simulink model "modelofisicocompleto"  (R2017a)
settings: Solver=FixedStepAuto  StartTime=0.0  StopTime=inf  FixedStep=1e-3  MaxStep=1e-3  RelTol=1e-3
undefined symbols (not defined in the file): bac, baiz, bcx, bcy, Beqtran, Bheqd, bw, g, Kcy, ksac, ksaiz, ksiac, ksiaiz, Kw, lh0, Meq, Mheq, Rd, Rr, rt, rtd, tau, xl0, xt0, yl0, yt0
libraries: simulink x3, powerlib_meascontrol x2, vrlib x1
settings Model: SimulationMode=accelerator  Creator=tomas  LastModifiedBy=tomas
settings HardwareCC: ProdBitPerPointer=32  ProdBitPerSizeT=32  ProdBitPerPtrDiffT=32  ProdWordSize=32  ProdHWDeviceType=Intel->x86-32 (Windows32)

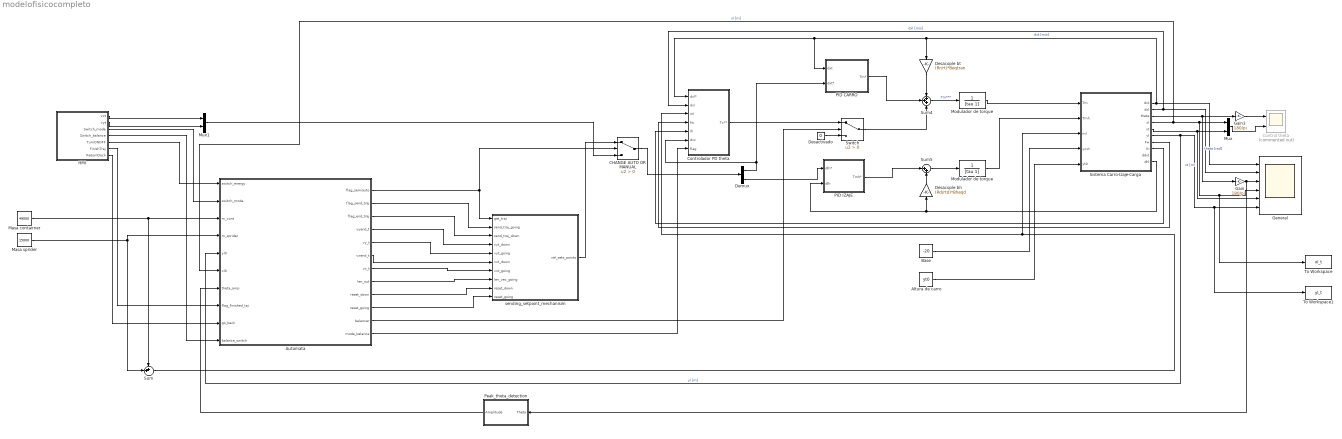
== system modelofisicocompleto ==
  Altura de carro : Constant  Value=yt0
  Automata : Stateflow chart  TreatAsAtomicUnit=on
  "Base " : Constant  Value=-20
  CHANGE AUTO OR MANUAL : Switch  Criteria=u2 > Threshold
  Control theta : Scope  Commented=on  NumInputPorts=2
  Controlador PD theta : Subsystem
  Demux : Demux  Outputs=2
  Desacople bh : Gain  Gain=(Rd/rtd)*Bheqd
  Desacople bt : Gain  Gain=(Rr/rt)*Beqtran
  Desactivado : Constant  Value=0
  Gain : Gain  Gain=180/pi
  Gain3 : Gain  Gain=180/pi
  General : Scope  NumInputPorts=6
  HMI : Subsystem
  Masa contairner : Constant  Value=49000
  Masa sprider : Constant  Value=15000
  Modulador de torque : TransferFcn  Denominator=[tau 1]
  "Modulador de torque  " : TransferFcn  Denominator=[tau 1]
  Mux : Mux  Inputs=2
  Mux1 : Mux  Inputs=2
  "PID CARRO " : Subsystem
  PID IZAJE : Subsystem
  Peak_theta_detection : Subsystem
  "Sistema Carro-Izaje-Carga " : Subsystem
  Sum : Sum  Inputs=++|
  Sum4 : Sum  Inputs=+++
  Sum5 : Sum  Inputs=|++
  Switch : Switch  Criteria=u2 > Threshold
  To Workspace : ToWorkspace  VariableName=xl_t  SampleTime=-1
  To Workspace1 : ToWorkspace  VariableName=yl_t  SampleTime=-1
  sending_setpoint_mechanisim : Subsystem
  wires:
  Sum4/1 -> "Modulador de torque  "/1  "Tm***"
  Desacople bt/1 -> Sum4/1
  Sum5/1 -> Modulador de torque/1
  Desacople bh/1 -> Sum5/2
  PID IZAJE/1("Tmh* ") -> Sum5/1
  Switch/1 -> Sum4/3
  Modulador de torque/1 -> "Sistema Carro-Izaje-Carga "/2(Tmh)
  "Base "/1 -> "Sistema Carro-Izaje-Carga "/4(ycxt)
  Altura de carro/1 -> "Sistema Carro-Izaje-Carga "/5(yt0)
  "Sistema Carro-Izaje-Carga "/1(dxt) -> Controlador PD theta/1(dxl*), "PID CARRO "/1(dxt), Desacople bt/1, General/1  "dxt [m/s]"
  "Sistema Carro-Izaje-Carga "/10(dhl) -> PID IZAJE/2(dlh), Desacople bh/1
  Controlador PD theta/1(Tc**) -> Switch/1
  Desactivado/1 -> Switch/3
  "Sistema Carro-Izaje-Carga "/8(lh) -> Controlador PD theta/5(lh)
  "Sistema Carro-Izaje-Carga "/7(Fw) -> Controlador PD theta/4(fw)
  Sum/1 -> Controlador PD theta/3(ml), "Sistema Carro-Izaje-Carga "/3(ml)
  "Sistema Carro-Izaje-Carga "/2(dxl) -> Controlador PD theta/2(dxl), General/2  "dxl [m/s]"
  Mux/1 -> Control theta/2
  "Sistema Carro-Izaje-Carga "/3(theta) -> Gain/1, Gain3/1  "theta [rad]"
  "Sistema Carro-Izaje-Carga "/4(xl) -> Automata/6(xl0), To Workspace/1, General/4, Mux/1  "xl [m]"
  "Sistema Carro-Izaje-Carga "/5(xt) -> General/5, Mux/2  "xt [m]"
  "Sistema Carro-Izaje-Carga "/6(yl) -> Automata/5(yl0), To Workspace1/1, General/6  "yl [m]"
  "Modulador de torque  "/1 -> "Sistema Carro-Izaje-Carga "/1(Tm)
  "PID CARRO "/1(Tm*) -> Sum4/2
  Gain/1 -> Peak_theta_detection/1(Theta), General/3
  Masa sprider/1 -> Automata/4(m_sprider), Sum/2
  Masa contairner/1 -> Sum/1, Automata/3(m_cont)
  Gain3/1 -> Control theta/1
  Automata/11(balancer) -> Switch/2
  HMI/4(Switch_balance) -> Automata/10(balance_switch)
  HMI/3(Switch_mode) -> Automata/2(switch_mode)
  HMI/1(vxt) -> Mux1/1
  HMI/2(vyt) -> Mux1/2
  Automata/1(flag_semiauto) -> CHANGE AUTO OR MANUAL/2, sending_setpoint_mechanisim/1(get_traj)
  CHANGE AUTO OR MANUAL/1 -> Demux/1
  Demux/1 -> Controlador PD theta/6(dxc), "PID CARRO "/2(dxt*)
  Demux/2 -> PID IZAJE/1(dlh*)
  Peak_theta_detection/1(Amplitude) -> Automata/7(theta_amp)
  Mux1/1 -> CHANGE AUTO OR MANUAL/3
  HMI/5(TurnONOFF) -> Automata/1(switch_energy)
  HMI/6(FinishTraj) -> Automata/8(flag_finished_taj)
  HMI/7(ReturnDock) -> Automata/9(go_back)
  Automata/2(flag_send_traj) -> sending_setpoint_mechanisim/2(send_traj_going)
  Automata/3(flag_end_traj) -> sending_setpoint_mechanisim/3(send_traj_down)
  sending_setpoint_mechanisim/1(vel_sets_points) -> CHANGE AUTO OR MANUAL/1
  Automata/7(vx_t) -> sending_setpoint_mechanisim/7(vxt_going)
  Automata/5(vy_t) -> sending_setpoint_mechanisim/5(vyt_going)
  Automata/4(vyend_t) -> sending_setpoint_mechanisim/4(vyt_down)
  Automata/6(vxend_t) -> sending_setpoint_mechanisim/6(vxt_down)
  Automata/8(len_out) -> sending_setpoint_mechanisim/8(len_vec_going)
  Automata/10(reset_going) -> sending_setpoint_mechanisim/10(reset_going)
  Automata/9(reset_down) -> sending_setpoint_mechanisim/9(reset_down)
  Automata/12(mode_balance) -> Controlador PD theta/7("flag ")

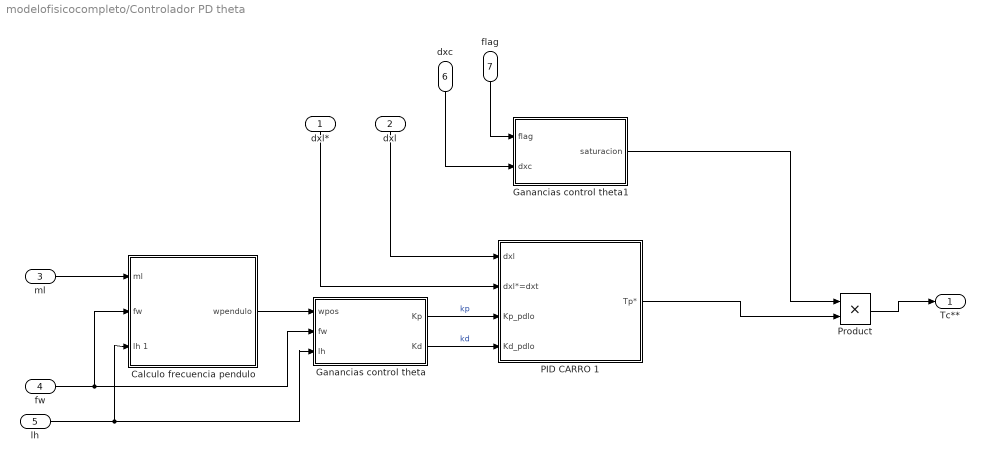
== system modelofisicocompleto/Controlador PD theta ==
  dxl* : Inport
  dxl : Inport  Port=2
  ml : Inport  Port=3
  fw : Inport  Port=4
  lh : Inport  Port=5
  dxc : Inport  Port=6
  "flag " : Inport  Port=7
  Calculo frecuencia pendulo : Subsystem
  Ganancias control theta : MATLAB Function  TreatAsAtomicUnit=on
  Ganancias control theta1 : MATLAB Function  TreatAsAtomicUnit=on
  PID CARRO 1 : Subsystem
  Product : Product
  Tc** : Outport
  wires:
  Calculo frecuencia pendulo/1("wpendulo ") -> Ganancias control theta/1(wpos)
  ml/1 -> Calculo frecuencia pendulo/1("ml ")
  Ganancias control theta/1(Kp) -> PID CARRO 1/3(Kp_pdlo)  "kp"
  Ganancias control theta/2(Kd) -> PID CARRO 1/4(Kd_pdlo)  "kd"
  dxl/1 -> PID CARRO 1/1(dxl)
  lh/1 -> Calculo frecuencia pendulo/3(lh 1), Ganancias control theta/3(lh)
  fw/1 -> Calculo frecuencia pendulo/2("fw "), Ganancias control theta/2(fw)
  dxl*/1 -> PID CARRO 1/2(dxl*=dxt)
  PID CARRO 1/1(Tp*) -> Product/2
  dxc/1 -> Ganancias control theta1/2(dxc)
  Ganancias control theta1/1(saturacion) -> Product/1
  Product/1 -> Tc**/1
  "flag "/1 -> Ganancias control theta1/1(flag)

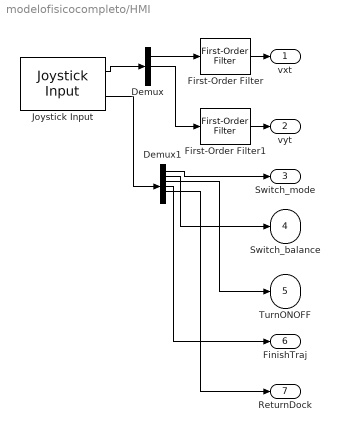
== system modelofisicocompleto/HMI ==
  Demux : Demux  Outputs=3
  Demux1 : Demux  Outputs=6
  First-Order Filter : powerlib_meascontrol/Filters/First-Order Filter  FilterType=Lowpass  Tc=10e-3  Ts=0  Initialize=off  Vac_Init=[0, 0, 60]  Vdc_Init=0  PlotResponse=off  FreqRange="[0,  200,  1]"
      settings: SourceProductName=Simscape Power Systems
  First-Order Filter1 : powerlib_meascontrol/Filters/First-Order Filter  FilterType=Lowpass  Tc=10e-3  Ts=0  Initialize=off  Vac_Init=[0, 0, 60]  Vdc_Init=0  PlotResponse=off  FreqRange="[0,  200,  1]"
      settings: SourceProductName=Simscape Power Systems
  Joystick Input : vrlib/Joystick Input  joyid=1  adjustports=on  forcefeed=off
      settings: SourceProductBaseCode=VR
  vxt : Outport
  vyt : Outport  Port=2
  Switch_mode : Outport  Port=3
  Switch_balance : Outport  Port=4
  TurnONOFF : Outport  Port=5
  FinishTraj : Outport  Port=6
  ReturnDock : Outport  Port=7
  wires:
  First-Order Filter1/1 -> vyt/1
  First-Order Filter/1 -> vxt/1
  Demux1/2 -> Switch_balance/1
  Joystick Input/2 -> Demux1/1
  Demux1/1 -> Switch_mode/1
  Joystick Input/1 -> Demux/1
  Demux/1 -> First-Order Filter/1
  Demux/2 -> First-Order Filter1/1
  Demux1/3 -> TurnONOFF/1
  Demux1/4 -> FinishTraj/1
  Demux1/5 -> ReturnDock/1

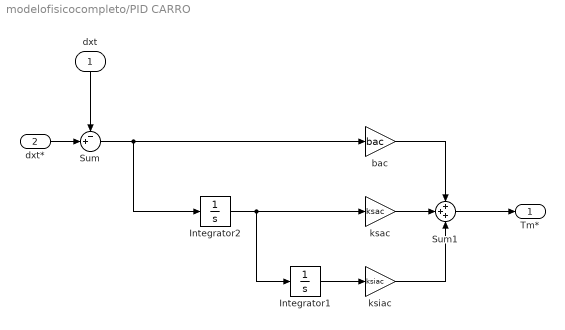
== system modelofisicocompleto/PID CARRO  ==
  dxt : Inport
  dxt* : Inport  Port=2
  Integrator1 : Integrator
  Integrator2 : Integrator
  Sum : Sum  Inputs=-+|
  Sum1 : Sum  Inputs=+++
  bac : Gain  Gain=bac
  ksac : Gain  Gain=ksac
  ksiac : Gain  Gain=ksiac
  Tm* : Outport
  wires:
  dxt*/1 -> Sum/2
  dxt/1 -> Sum/1
  Sum1/1 -> Tm*/1
  bac/1 -> Sum1/1
  ksac/1 -> Sum1/2
  Integrator1/1 -> ksiac/1
  ksiac/1 -> Sum1/3
  Sum/1 -> bac/1, Integrator2/1
  Integrator2/1 -> Integrator1/1, ksac/1

== system modelofisicocompleto/PID IZAJE ==
  dlh* : Inport
  dlh : Inport  Port=2
  Integrator1 : Integrator
  Integrator2 : Integrator
  Sum2 : Sum  Inputs=|+-
  Sum3 : Sum  Inputs=+++
  baiz : Gain  Gain=baiz
  ksaiz : Gain  Gain=ksaiz
  ksiaiz : Gain  Gain=ksiaiz
  "Tmh* " : Outport
  wires:
  dlh/1 -> Sum2/2
  Sum3/1 -> "Tmh* "/1
  ksaiz/1 -> Sum3/2
  Integrator1/1 -> ksiaiz/1
  baiz/1 -> Sum3/1
  ksiaiz/1 -> Sum3/3
  dlh*/1 -> Sum2/1
  Sum2/1 -> baiz/1, Integrator2/1
  Integrator2/1 -> Integrator1/1, ksaiz/1

== system modelofisicocompleto/Peak_theta_detection ==
  Theta : Inport
  Detect Decrease : simulink/Logic and Bit Operations/Detect Decrease  vinit=0.0  OutDataTypeStr=boolean
  Detect Rise Positive : simulink/Logic and Bit Operations/Detect Rise Positive  vinit=0  OutDataTypeStr=boolean
  MinMax Running Resettable : simulink/Math Operations/MinMax Running Resettable  Function=max  vinit=0.0
  Subsystem : Subsystem
  Amplitude : Outport
  wires:
  Theta/1 -> Detect Decrease/1, Detect Rise Positive/1, MinMax Running Resettable/1
  Subsystem/1(Out1) -> Amplitude/1
  MinMax Running Resettable/1 -> Subsystem/1(In1)
  Detect Rise Positive/1 -> MinMax Running Resettable/2
  Detect Decrease/1 -> Subsystem/Trigger

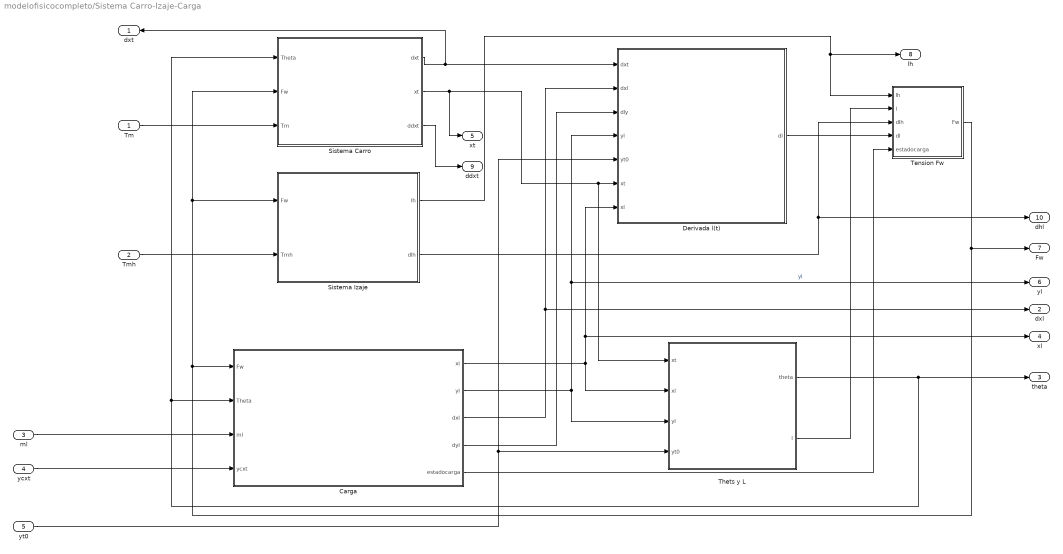
== system modelofisicocompleto/Sistema Carro-Izaje-Carga  ==
  Tm : Inport
  Tmh : Inport  Port=2
  ml : Inport  Port=3
  ycxt : Inport  Port=4
  yt0 : Inport  Port=5
  "Carga " : Subsystem
  Derivada l(t) : Subsystem
  Sistema Carro : Subsystem
  Sistema Izaje : Subsystem
  Tension Fw : Subsystem
  Thets y L : Subsystem
  dxt : Outport
  dxl : Outport  Port=2
  theta : Outport  Port=3
  xl : Outport  Port=4
  xt : Outport  Port=5
  yl : Outport  Port=6
  Fw : Outport  Port=7
  lh : Outport  Port=8
  ddxt : Outport  Port=9
  dhl : Outport  Port=10
  wires:
  Sistema Carro/2(xt) -> xt/1, Derivada l(t)/6(xt), Thets y L/1(xt)
  Sistema Carro/1("dxt ") -> dxt/1, Derivada l(t)/1(dxt)
  Sistema Izaje/1(lh) -> lh/1, Tension Fw/1(lh)
  Sistema Izaje/2(dlh) -> dhl/1, Tension Fw/3(dlh)
  "Carga "/2(yl) -> yl/1, Derivada l(t)/4(yl), Thets y L/3(yl)  "yl"
  "Carga "/3(dxl) -> dxl/1, Derivada l(t)/2(dxl)
  "Carga "/4(dyl) -> Derivada l(t)/3(dly)
  Derivada l(t)/1(dl) -> Tension Fw/4(dl)
  Thets y L/1("theta ") -> theta/1, Sistema Carro/1(Theta), "Carga "/2(Theta)
  ml/1 -> "Carga "/3(ml)
  ycxt/1 -> "Carga "/4(ycxt)
  "Carga "/5("estadocarga ") -> Tension Fw/5(estadocarga)
  Thets y L/2("l ") -> Tension Fw/2(l)
  Tm/1 -> Sistema Carro/3(Tm)
  Tmh/1 -> Sistema Izaje/2(Tmh)
  yt0/1 -> Derivada l(t)/5(yt0), Thets y L/4(yt0)
  "Carga "/1(xl) -> Derivada l(t)/7(xl), xl/1, Thets y L/2(xl)
  Tension Fw/1("Fw ") -> Fw/1, Sistema Carro/2(Fw), Sistema Izaje/1(Fw), "Carga "/1(Fw)
  Sistema Carro/3("ddxt ") -> ddxt/1

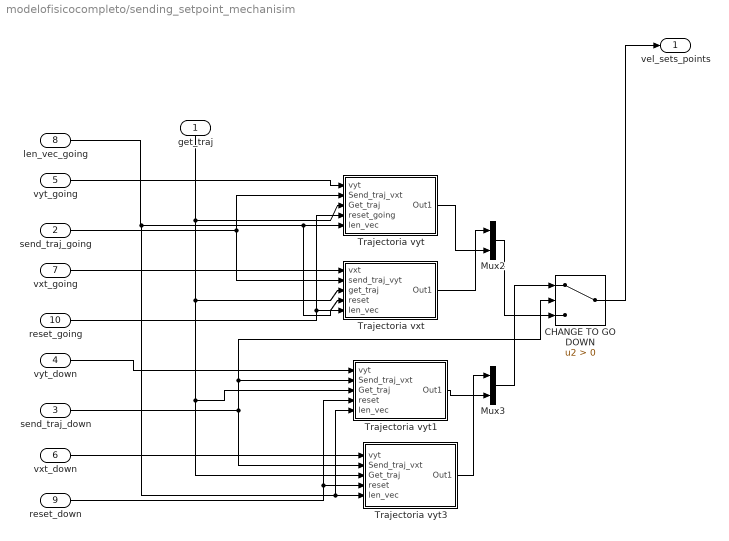
== system modelofisicocompleto/sending_setpoint_mechanisim ==
  get_traj : Inport
  send_traj_going : Inport  Port=2
  send_traj_down : Inport  Port=3
  vyt_down : Inport  Port=4
  vyt_going : Inport  Port=5
  vxt_down : Inport  Port=6
  vxt_going : Inport  Port=7
  len_vec_going : Inport  Port=8
  reset_down : Inport  Port=9
  reset_going : Inport  Port=10
  CHANGE TO GO DOWN : Switch  Criteria=u2 > Threshold
  Mux2 : Mux  Inputs=2
  Mux3 : Mux  Inputs=2
  Trajectoria vxt : Subsystem
  Trajectoria vyt : Subsystem
  Trajectoria vyt1 : Subsystem
  Trajectoria vyt3 : Subsystem
  vel_sets_points : Outport
  wires:
  get_traj/1 -> Trajectoria vyt3/3(Get_traj), Trajectoria vyt1/3(Get_traj), Trajectoria vxt/3("get_traj "), Trajectoria vyt/3(Get_traj)
  vyt_going/1 -> Trajectoria vyt/1("vyt ")
  Trajectoria vxt/1(Out1) -> Mux2/1
  Trajectoria vyt/1(Out1) -> Mux2/2
  vxt_going/1 -> Trajectoria vxt/1(vxt)
  send_traj_going/1 -> Trajectoria vxt/2(send_traj_vyt), Trajectoria vyt/2("Send_traj_vxt ")
  vyt_down/1 -> Trajectoria vyt1/1("vyt ")
  vxt_down/1 -> Trajectoria vyt3/1("vyt ")
  send_traj_down/1 -> Trajectoria vyt3/2("Send_traj_vxt "), Trajectoria vyt1/2("Send_traj_vxt "), CHANGE TO GO DOWN/2
  Trajectoria vyt1/1(Out1) -> Mux3/2
  Trajectoria vyt3/1(Out1) -> Mux3/1
  CHANGE TO GO DOWN/1 -> vel_sets_points/1
  Mux3/1 -> CHANGE TO GO DOWN/1
  Mux2/1 -> CHANGE TO GO DOWN/3
  reset_going/1 -> Trajectoria vxt/4(reset), Trajectoria vyt/4(reset_going)
  reset_down/1 -> Trajectoria vyt3/4(reset), Trajectoria vyt1/4(reset)
  len_vec_going/1 -> Trajectoria vyt3/5(len_vec), Trajectoria vyt1/5(len_vec), Trajectoria vxt/5(len_vec), Trajectoria vyt/5(len_vec)

== system modelofisicocompleto/Controlador PD theta/Calculo frecuencia pendulo ==
  "ml " : Inport
  "fw " : Inport  Port=2
  lh 1 : Inport  Port=3
  Abs : Abs
  Divide : Product  Inputs=*/
  Gain : Gain  Gain=80
  Product : Product
  Sqrt : Sqrt  OutputSignalType=complex  SaturateOnIntegerOverflow=on
  "wpendulo " : Outport
  wires:
  "fw "/1 -> Divide/1
  Divide/1 -> Sqrt/1
  lh 1/1 -> Product/2
  Product/1 -> Divide/2
  Sqrt/1 -> Abs/1
  "ml "/1 -> Product/1
  Abs/1 -> Gain/1
  Gain/1 -> "wpendulo "/1

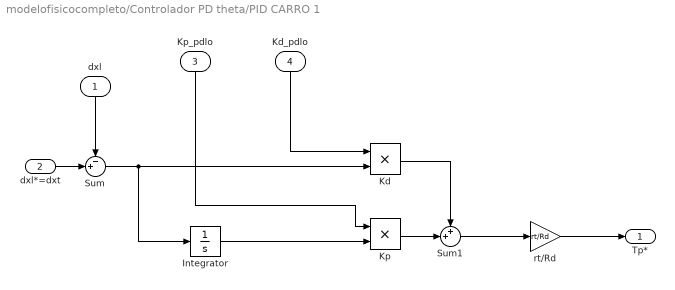
== system modelofisicocompleto/Controlador PD theta/PID CARRO 1 ==
  dxl : Inport
  dxl*=dxt : Inport  Port=2
  Kp_pdlo : Inport  Port=3
  Kd_pdlo : Inport  Port=4
  Integrator : Integrator
  Kd : Product
  Kp : Product
  Sum : Sum  Inputs=-+|
  Sum1 : Sum  Inputs=++|
  rt/Rd : Gain  Gain=rt/Rd
  Tp* : Outport
  wires:
  dxl*=dxt/1 -> Sum/2
  dxl/1 -> Sum/1
  Sum1/1 -> rt/Rd/1
  Sum/1 -> Integrator/1, Kd/2
  Kd/1 -> Sum1/1
  Integrator/1 -> Kp/2
  Kp/1 -> Sum1/2
  Kp_pdlo/1 -> Kp/1
  Kd_pdlo/1 -> Kd/1
  rt/Rd/1 -> Tp*/1

== system modelofisicocompleto/Peak_theta_detection/Subsystem ==
  In1 : Inport
  Trigger : TriggerPort  VariantControl=Variant  PortDimensions=1
  Out1 : Outport
  wires:
  In1/1 -> Out1/1

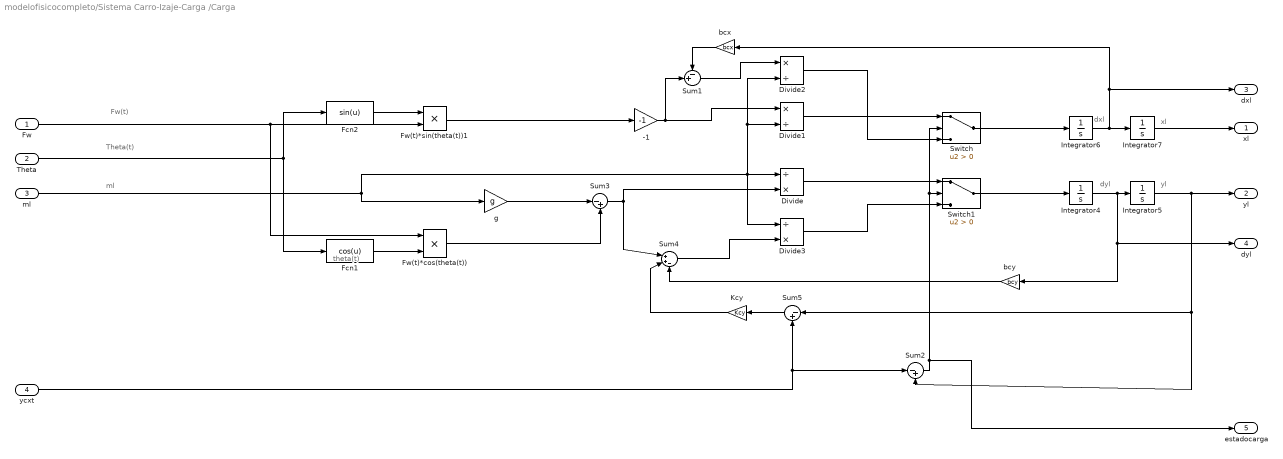
== system modelofisicocompleto/Sistema Carro-Izaje-Carga /Carga  ==
  note: Theta(t)
  note: Fw(t)
  note: ml
  note: theta(t)
  note: dyl
  note: yl
  note: dxl
  note: xl
  Fw : Inport
  Theta : Inport  Port=2
  ml : Inport  Port=3
  ycxt : Inport  Port=4
  -1 : Gain  Gain=-1
  Divide : Product  Inputs=/*
  Divide1 : Product  Inputs=*/
  Divide2 : Product  Inputs=*/
  Divide3 : Product  Inputs=/*
  Fcn1 : Fcn  Expr=cos(u)
  Fcn2 : Fcn  Expr=sin(u)
  Fw(t)*cos(theta(t)) : Product
  Fw(t)*sin(theta(t))1 : Product
  Integrator4 : Integrator
  Integrator5 : Integrator  InitialCondition=yl0
  Integrator6 : Integrator
  Integrator7 : Integrator  InitialCondition=xl0
  Kcy : Gain  Gain=Kcy
  Sum1 : Sum  Inputs=-+|
  Sum2 : Sum  Inputs=|-+
  Sum3 : Sum  Inputs=|-+
  Sum4 : Sum  Inputs=|++-
  Sum5 : Sum  Inputs=|-+
  Switch : Switch  Criteria=u2 > Threshold
  Switch1 : Switch  Criteria=u2 > Threshold
  bcx : Gain  Gain=bcx
  bcy : Gain  Gain=bcy
  g : Gain  Gain=g
  xl : Outport
  yl : Outport  Port=2
  dxl : Outport  Port=3
  dyl : Outport  Port=4
  "estadocarga " : Outport  Port=5
  wires:
  Fcn2/1 -> Fw(t)*sin(theta(t))1/1
  Theta/1 -> Fcn1/1, Fcn2/1
  g/1 -> Sum3/1
  Fcn1/1 -> Fw(t)*cos(theta(t))/2
  Fw(t)*cos(theta(t))/1 -> Sum3/2
  Fw/1 -> Fw(t)*cos(theta(t))/1, Fw(t)*sin(theta(t))1/2
  ml/1 -> Divide1/2, Divide2/2, Divide3/1, Divide/1, g/1
  Integrator7/1 -> xl/1
  Integrator6/1 -> Integrator7/1, dxl/1, bcx/1
  Fw(t)*sin(theta(t))1/1 -> -1/1
  Integrator5/1 -> Sum2/2, Sum5/1, yl/1
  Divide1/1 -> Switch/1
  -1/1 -> Sum1/2, Divide1/1
  Integrator4/1 -> dyl/1, bcy/1, Integrator5/1
  Sum3/1 -> Sum4/1, Divide/2
  Switch/1 -> Integrator6/1
  bcx/1 -> Sum1/1
  Sum2/1 -> "estadocarga "/1, Switch1/2, Switch/2
  ycxt/1 -> Sum2/1, Sum5/2
  Sum1/1 -> Divide2/1
  Divide2/1 -> Switch/3
  Sum4/1 -> Divide3/2
  Divide3/1 -> Switch1/3
  Switch1/1 -> Integrator4/1
  Divide/1 -> Switch1/1
  Sum5/1 -> Kcy/1
  Kcy/1 -> Sum4/2
  bcy/1 -> Sum4/3

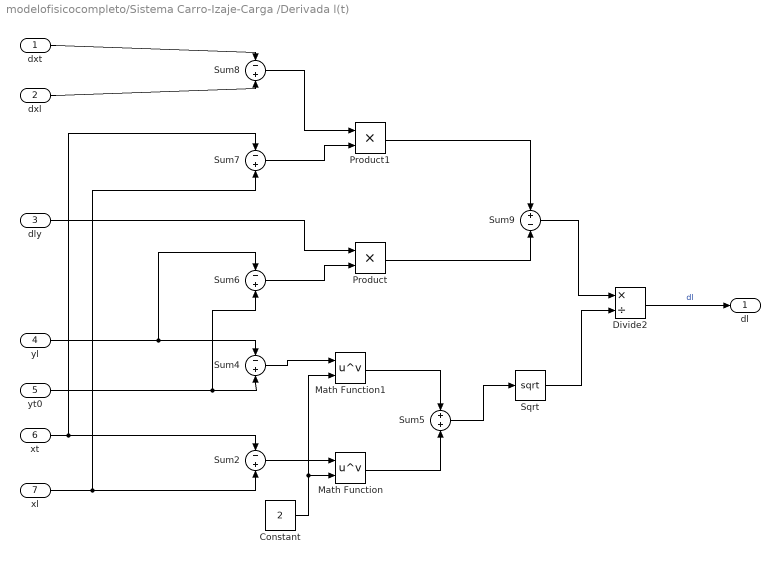
== system modelofisicocompleto/Sistema Carro-Izaje-Carga /Derivada l(t) ==
  dxt : Inport
  dxl : Inport  Port=2
  dly : Inport  Port=3
  yl : Inport  Port=4
  yt0 : Inport  Port=5
  xt : Inport  Port=6
  xl : Inport  Port=7
  Constant : Constant  Value=2
  Divide2 : Product  Inputs=*/
  Math Function : Math  Operator=pow  SaturateOnIntegerOverflow=on
  Math Function1 : Math  Operator=pow  SaturateOnIntegerOverflow=on
  Product : Product
  Product1 : Product
  Sqrt : Sqrt  SaturateOnIntegerOverflow=on
  Sum{2,4,6..8} (5 alike) : Sum  Inputs=-+
  Sum5 : Sum
  Sum9 : Sum  Inputs=+-
  dl : Outport
  wires:
  Divide2/1 -> dl/1  "dl"
  dly/1 -> Product/1
  yl/1 -> Sum6/1, Sum4/1
  xl/1 -> Sum7/2, Sum2/2
  Product/1 -> Sum9/2
  dxt/1 -> Sum8/1
  Sum5/1 -> Sqrt/1
  Constant/1 -> Math Function1/2, Math Function/2
  yt0/1 -> Sum4/2, Sum6/2
  dxl/1 -> Sum8/2
  Math Function1/1 -> Sum5/1
  Sum8/1 -> Product1/1
  Sum9/1 -> Divide2/1
  Math Function/1 -> Sum5/2
  xt/1 -> Sum7/1, Sum2/1
  Sum6/1 -> Product/2
  Sum7/1 -> Product1/2
  Product1/1 -> Sum9/1
  Sum4/1 -> Math Function1/1
  Sqrt/1 -> Divide2/2
  Sum2/1 -> Math Function/1

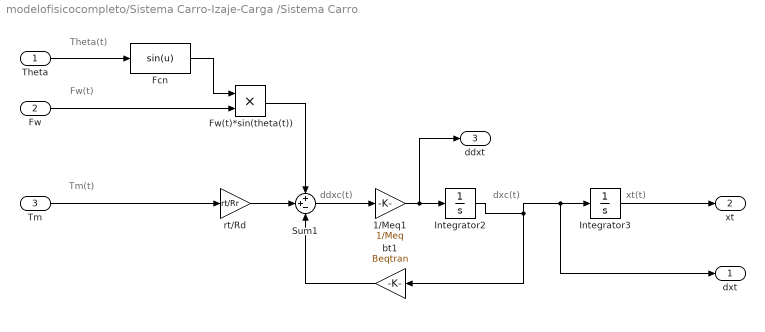
== system modelofisicocompleto/Sistema Carro-Izaje-Carga /Sistema Carro ==
  note: dxc(t)
  note: xt(t)
  note: ddxc(t)
  note: Theta(t)
  note: Fw(t)
  note: Tm(t)
  Theta : Inport
  Fw : Inport  Port=2
  Tm : Inport  Port=3
  1/Meq1 : Gain  Gain=1/Meq
  Fcn : Fcn  Expr=sin(u)
  Fw(t)*sin(theta(t)) : Product
  Integrator2 : Integrator
  Integrator3 : Integrator  InitialCondition=xt0
  Sum1 : Sum  Inputs=++-
  bt1 : Gain  Gain=Beqtran
  rt/Rd : Gain  Gain=rt/Rr
  "dxt " : Outport
  xt : Outport  Port=2
  "ddxt " : Outport  Port=3
  wires:
  Integrator3/1 -> xt/1
  Sum1/1 -> 1/Meq1/1
  Fw/1 -> Fw(t)*sin(theta(t))/2
  Fcn/1 -> Fw(t)*sin(theta(t))/1
  rt/Rd/1 -> Sum1/2
  Theta/1 -> Fcn/1
  Fw(t)*sin(theta(t))/1 -> Sum1/1
  1/Meq1/1 -> "ddxt "/1, Integrator2/1
  Tm/1 -> rt/Rd/1
  bt1/1 -> Sum1/3
  Integrator2/1 -> "dxt "/1, Integrator3/1, bt1/1

== system modelofisicocompleto/Sistema Carro-Izaje-Carga /Sistema Izaje ==
  note: lh(t)
  note: dlh(t)
  note: ddlh(t)
  note: Tmh(t)
  note: Fw(t)
  Fw : Inport
  Tmh : Inport  Port=2
  1/Meq : Gain  Gain=1/Mheq
  Integrator : Integrator
  Integrator1 : Integrator  InitialCondition=lh0
  Sum : Sum  Inputs=++-
  bt : Gain  Gain=Bheqd
  rtd/Rd : Gain  Gain=-rtd/Rd
  lh : Outport
  dlh : Outport  Port=2
  wires:
  Integrator/1 -> dlh/1, bt/1, Integrator1/1
  Integrator1/1 -> lh/1
  rtd/Rd/1 -> Sum/2
  bt/1 -> Sum/3
  Fw/1 -> Sum/1
  Tmh/1 -> rtd/Rd/1
  1/Meq/1 -> Integrator/1
  Sum/1 -> 1/Meq/1

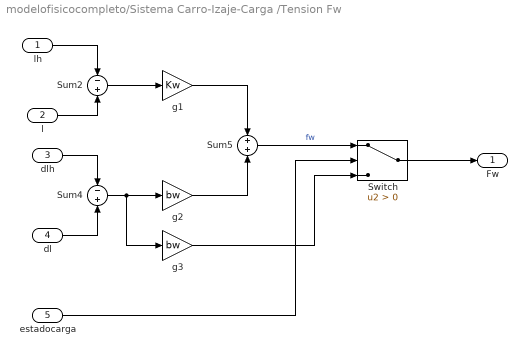
== system modelofisicocompleto/Sistema Carro-Izaje-Carga /Tension Fw ==
  lh : Inport
  l : Inport  Port=2
  dlh : Inport  Port=3
  dl : Inport  Port=4
  estadocarga : Inport  Port=5
  Sum2 : Sum  Inputs=-+
  Sum4 : Sum  Inputs=-+
  Sum5 : Sum
  Switch : Switch  Criteria=u2 > Threshold
  g1 : Gain  Gain=Kw
  g2 : Gain  Gain=bw
  g3 : Gain  Gain=bw
  "Fw " : Outport
  wires:
  l/1 -> Sum2/2
  lh/1 -> Sum2/1
  dl/1 -> Sum4/2
  g2/1 -> Sum5/2
  Sum5/1 -> Switch/1  "fw"
  Sum4/1 -> g3/1, g2/1
  g1/1 -> Sum5/1
  dlh/1 -> Sum4/1
  Sum2/1 -> g1/1
  Switch/1 -> "Fw "/1
  estadocarga/1 -> Switch/2
  g3/1 -> Switch/3

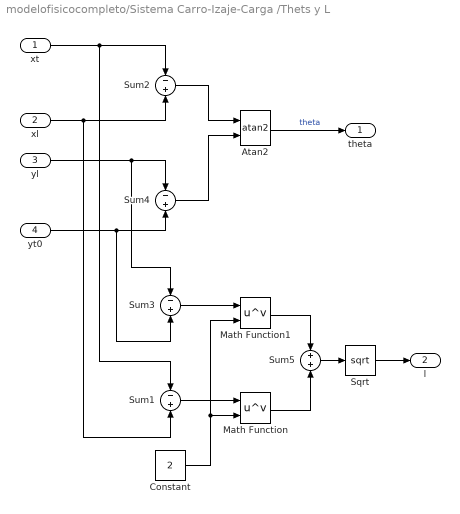
== system modelofisicocompleto/Sistema Carro-Izaje-Carga /Thets y L ==
  xt : Inport
  xl : Inport  Port=2
  yl : Inport  Port=3
  yt0 : Inport  Port=4
  Atan2 : Trigonometry  Operator=atan2
  Constant : Constant  Value=2
  Math Function : Math  Operator=pow  SaturateOnIntegerOverflow=on
  Math Function1 : Math  Operator=pow  SaturateOnIntegerOverflow=on
  Sqrt : Sqrt  SaturateOnIntegerOverflow=on
  Sum{1..4} (4 alike) : Sum  Inputs=-+
  Sum5 : Sum
  "theta " : Outport
  "l " : Outport  Port=2
  wires:
  Sum4/1 -> Atan2/2
  xt/1 -> Sum1/1, Sum2/1
  xl/1 -> Sum1/2, Sum2/2
  yt0/1 -> Sum3/2, Sum4/2
  Atan2/1 -> "theta "/1  "theta"
  yl/1 -> Sum3/1, Sum4/1
  Sum2/1 -> Atan2/1
  Sqrt/1 -> "l "/1
  Math Function/1 -> Sum5/2
  Math Function1/1 -> Sum5/1
  Sum3/1 -> Math Function1/1
  Sum1/1 -> Math Function/1
  Constant/1 -> Math Function/2, Math Function1/2
  Sum5/1 -> Sqrt/1

== system modelofisicocompleto/sending_setpoint_mechanisim/Trajectoria vxt ==
  vxt : Inport
  send_traj_vyt : Inport  Port=2
  "get_traj " : Inport  Port=3
  reset : Inport  Port=4
  len_vec : Inport  Port=5
  Subsystem2 : Subsystem
  Subsystem3 : Subsystem
  Out1 : Outport
  wires:
  vxt/1 -> Subsystem2/1(In1)
  Subsystem2/1(Out1) -> Subsystem3/1(In1)
  send_traj_vyt/1 -> Subsystem3/Enable
  Subsystem3/1(Out1) -> Out1/1
  "get_traj "/1 -> Subsystem2/Enable
  reset/1 -> Subsystem3/2(In2)
  len_vec/1 -> Subsystem3/3(In3)

== system modelofisicocompleto/sending_setpoint_mechanisim/Trajectoria vyt ==
  "vyt " : Inport
  "Send_traj_vxt " : Inport  Port=2
  Get_traj : Inport  Port=3
  reset_going : Inport  Port=4
  len_vec : Inport  Port=5
  Subsystem2 : Subsystem
  Subsystem3 : Subsystem
  Out1 : Outport
  wires:
  "vyt "/1 -> Subsystem2/1(In1)
  Subsystem2/1(Out1) -> Subsystem3/1(In1)
  "Send_traj_vxt "/1 -> Subsystem3/Enable
  Subsystem3/1(Out1) -> Out1/1
  Get_traj/1 -> Subsystem2/Enable
  reset_going/1 -> Subsystem3/2(In2)
  len_vec/1 -> Subsystem3/3(In3)

== system modelofisicocompleto/sending_setpoint_mechanisim/Trajectoria vyt1 ==
  "vyt " : Inport
  "Send_traj_vxt " : Inport  Port=2
  Get_traj : Inport  Port=3
  reset : Inport  Port=4
  len_vec : Inport  Port=5
  Subsystem2 : Subsystem
  Subsystem3 : Subsystem
  Out1 : Outport
  wires:
  "vyt "/1 -> Subsystem2/1(In1)
  Subsystem2/1(Out1) -> Subsystem3/1(In1)
  "Send_traj_vxt "/1 -> Subsystem3/Enable
  Subsystem3/1(Out1) -> Out1/1
  Get_traj/1 -> Subsystem2/Enable
  reset/1 -> Subsystem3/2(In2)
  len_vec/1 -> Subsystem3/3(In3)

== system modelofisicocompleto/sending_setpoint_mechanisim/Trajectoria vyt3 ==
  "vyt " : Inport
  "Send_traj_vxt " : Inport  Port=2
  Get_traj : Inport  Port=3
  reset : Inport  Port=4
  len_vec : Inport  Port=5
  Subsystem2 : Subsystem
  Subsystem3 : Subsystem
  Out1 : Outport
  wires:
  "vyt "/1 -> Subsystem2/1(In1)
  Subsystem2/1(Out1) -> Subsystem3/1(In1)
  "Send_traj_vxt "/1 -> Subsystem3/Enable
  Subsystem3/1(Out1) -> Out1/1
  Get_traj/1 -> Subsystem2/Enable
  reset/1 -> Subsystem3/2(In2)
  len_vec/1 -> Subsystem3/3(In3)

== system modelofisicocompleto/sending_setpoint_mechanisim/Trajectoria vxt/Subsystem2 ==
  In1 : Inport
  Enable : EnablePort
  Out1 : Outport
  wires:
  In1/1 -> Out1/1

== system modelofisicocompleto/sending_setpoint_mechanisim/Trajectoria vxt/Subsystem3 ==
  In1 : Inport
  In2 : Inport  Port=2
  In3 : Inport  Port=3
  Enable : EnablePort
  Resettable Subsystem : Subsystem  TreatAsAtomicUnit=on
  Out1 : Outport
  wires:
  In1/1 -> Resettable Subsystem/1(In1)
  In2/1 -> Resettable Subsystem/Reset
  Resettable Subsystem/1(Out1) -> Out1/1
  In3/1 -> Resettable Subsystem/2(len_vector)

== system modelofisicocompleto/sending_setpoint_mechanisim/Trajectoria vyt/Subsystem2 ==
  In1 : Inport
  Enable : EnablePort
  Out1 : Outport
  wires:
  In1/1 -> Out1/1

== system modelofisicocompleto/sending_setpoint_mechanisim/Trajectoria vyt/Subsystem3 ==
  In1 : Inport
  In2 : Inport  Port=2
  In3 : Inport  Port=3
  Enable : EnablePort
  Resettable Subsystem : Subsystem  TreatAsAtomicUnit=on
  Out1 : Outport
  wires:
  In1/1 -> Resettable Subsystem/1(In1)
  In2/1 -> Resettable Subsystem/Reset
  Resettable Subsystem/1(Out1) -> Out1/1
  In3/1 -> Resettable Subsystem/2(len_vector)

== system modelofisicocompleto/sending_setpoint_mechanisim/Trajectoria vyt1/Subsystem2 ==
  In1 : Inport
  Enable : EnablePort
  Out1 : Outport
  wires:
  In1/1 -> Out1/1

== system modelofisicocompleto/sending_setpoint_mechanisim/Trajectoria vyt1/Subsystem3 ==
  In1 : Inport
  In2 : Inport  Port=2
  In3 : Inport  Port=3
  Enable : EnablePort
  Resettable Subsystem : Subsystem  TreatAsAtomicUnit=on
  Out1 : Outport
  wires:
  In1/1 -> Resettable Subsystem/1(In1)
  In2/1 -> Resettable Subsystem/Reset
  Resettable Subsystem/1(Out1) -> Out1/1
  In3/1 -> Resettable Subsystem/2(len_vector)

== system modelofisicocompleto/sending_setpoint_mechanisim/Trajectoria vyt3/Subsystem2 ==
  In1 : Inport
  Enable : EnablePort
  Out1 : Outport
  wires:
  In1/1 -> Out1/1

== system modelofisicocompleto/sending_setpoint_mechanisim/Trajectoria vyt3/Subsystem3 ==
  In1 : Inport
  In2 : Inport  Port=2
  In3 : Inport  Port=3
  Enable : EnablePort
  Resettable Subsystem : Subsystem  TreatAsAtomicUnit=on
  Out1 : Outport
  wires:
  In1/1 -> Resettable Subsystem/1(In1)
  In2/1 -> Resettable Subsystem/Reset
  Resettable Subsystem/1(Out1) -> Out1/1
  In3/1 -> Resettable Subsystem/2(len_vector)

== system modelofisicocompleto/sending_setpoint_mechanisim/Trajectoria vxt/Subsystem3/Resettable Subsystem ==
  In1 : Inport
  len_vector : Inport  Port=2
  Reset : ResetPort  DisableCoverage=on  ResetTriggerType=either
  MATLAB Function : MATLAB Function  TreatAsAtomicUnit=on
  Memory : Memory
  Scope : Scope
  Out1 : Outport
  wires:
  len_vector/1 -> MATLAB Function/1(len_vec)
  MATLAB Function/2(vt) -> Out1/1
  MATLAB Function/1(cont) -> Scope/1, Memory/1
  Memory/1 -> MATLAB Function/3(cont_i)
  In1/1 -> MATLAB Function/2(qd)

== system modelofisicocompleto/sending_setpoint_mechanisim/Trajectoria vyt/Subsystem3/Resettable Subsystem ==
  In1 : Inport
  len_vector : Inport  Port=2
  Reset : ResetPort  DisableCoverage=on  ResetTriggerType=either
  MATLAB Function : MATLAB Function  TreatAsAtomicUnit=on
  Memory : Memory
  Out1 : Outport
  wires:
  In1/1 -> MATLAB Function/2(qd)
  MATLAB Function/2(vt) -> Out1/1
  Memory/1 -> MATLAB Function/3(cont_i)
  MATLAB Function/1(cont) -> Memory/1
  len_vector/1 -> MATLAB Function/1(len_vec)

== system modelofisicocompleto/sending_setpoint_mechanisim/Trajectoria vyt1/Subsystem3/Resettable Subsystem ==
  In1 : Inport
  len_vector : Inport  Port=2
  Reset : ResetPort  DisableCoverage=on  ResetTriggerType=either
  MATLAB Function : MATLAB Function  TreatAsAtomicUnit=on
  Memory : Memory
  Out1 : Outport
  wires:
  len_vector/1 -> MATLAB Function/1(len_vec)
  MATLAB Function/2(vt) -> Out1/1
  MATLAB Function/1(cont) -> Memory/1
  Memory/1 -> MATLAB Function/3(cont_i)
  In1/1 -> MATLAB Function/2(qd)

== system modelofisicocompleto/sending_setpoint_mechanisim/Trajectoria vyt3/Subsystem3/Resettable Subsystem ==
  In1 : Inport
  len_vector : Inport  Port=2
  Reset : ResetPort  DisableCoverage=on  ResetTriggerType=either
  MATLAB Function : MATLAB Function  TreatAsAtomicUnit=on
  Memory : Memory
  Out1 : Outport
  wires:
  len_vector/1 -> MATLAB Function/1(len_vec)
  MATLAB Function/2(vt) -> Out1/1
  MATLAB Function/1(cont) -> Memory/1
  Memory/1 -> MATLAB Function/3(cont_i)
  In1/1 -> MATLAB Function/2(qd)

== matlab function modelofisicocompleto/Controlador PD theta/Ganancias control theta1 ==
  data: flag input; dxc input; saturacion output
function saturacion  = fcn(flag,dxc)
    if(flag)
    if(abs(dxc)>0)
        saturacion =  0.8;
%     elseif(abs(dxc)>0.0001 && (ddxc==0))
%         saturacion =  0.7;
    else
        saturacion = 1.0;
    end
    else
    if(abs(dxc)>0)
        saturacion =  0.2;
%     elseif(abs(dxc)>0.0001 && (ddxc==0))
%         saturacion =  0.7;
    else
        saturacion = 0.6;
    end
    end
end

== matlab function modelofisicocompleto/Controlador PD theta/Ganancias control theta ==
  data: wpos input; Kp output; Kd output; fw input; lh input
function [Kp,Kd] = fcn(wpos,fw,lh)
    Meq=59008;
    Kp=wpos^2 + (fw/(Meq*lh));
    Kd=2*wpos;
end

== stateflow chart modelofisicocompleto/Automata ==
  state OFF
  state Sim_pulsadorONOFF1
  state Sim_pulsadorONOFF
  state ON
    state Level1
      state Deegre_Balancer [parallel]
        settings: executionOrder=1
        state OFF
          entry: balancer =0
        state Sim_pulsador
        state Sim_pulsador1
        state ON
          entry: balancer =1
        (default) -> ON.Level1.Deegre_Balancer.OFF
        Sim_pulsador -> ON.Level1.Deegre_Balancer.OFF : [balance_switch==0]
        ON.Level1.Deegre_Balancer.OFF -> Sim_pulsador1 : [balance_switch==1]
        ON.Level1.Deegre_Balancer.ON -> Sim_pulsador : [balance_switch==1]
        Sim_pulsador1 -> ON.Level1.Deegre_Balancer.ON : [balance_switch==0]
      state Operation_mode [parallel]
        settings: executionOrder=2
        state Automatic
          state Double_cycle
            entry: flag_semiauto = 1;
            flag_end_traj=0;
            flag_send_traj = 0;
            reset_going=0;
            reset_down=0;
            mode_balance = 1;
            state To_boat
              entry:  [vyt,vxt,xend,vx_end,vy_end,len] = gen_traj_boat([5,5,15,5,1,1],xl0,yl0,1,0,m_cont+m_sprider);
              vx_t=vxt; vy_t=vyt;vxend_t=vx_end;vyend_t=vy_end;len_out=len;
              state Go
                entry:
                flag_send_traj = 1;
              state Go_down
                entry:
                flag_send_traj = 1;
                flag_end_traj =1;
              state Finished
                entry:
                flag_end_traj=0;
                flag_send_traj = 0;
              (default) -> ON.Level1.Operation_mode.Automatic.Double_cycle.To_boat.Go
              ON.Level1.Operation_mode.Automatic.Double_cycle.To_boat.Go_down -> ON.Level1.Operation_mode.Automatic.Double_cycle.To_boat.Finished : [flag_finished_taj==1]
              ON.Level1.Operation_mode.Automatic.Double_cycle.To_boat.Go -> ON.Level1.Operation_mode.Automatic.Double_cycle.To_boat.Go_down : [(abs(xend-xl0) <= 0.05) && (theta_amp <= 0.5)]
            state container_to_container
              entry: mode_balance=0;
              [vyt,vxt,xend,vx_end,vy_end,len] = gen_traj_cont_cont([5,5,15,5,1,1],xl0,yl0,5,0);
              vx_t=vxt; vy_t=vyt;vxend_t=vx_end;vyend_t=vy_end;len_out=len;
              state Go_down
                entry:
                flag_send_traj = 1;
                flag_end_traj=1;
                reset_down =1;
              state Go
                entry:
                flag_send_traj = 1;
                reset_going=1;
              state Finished1
                entry:
                flag_end_traj=0;
                flag_send_traj = 0;
              (default) -> ON.Level1.Operation_mode.Automatic.Double_cycle.container_to_container.Go
              ON.Level1.Operation_mode.Automatic.Double_cycle.container_to_container.Go -> ON.Level1.Operation_mode.Automatic.Double_cycle.container_to_container.Go_down : [(abs(xend-xl0) <= 0.05) && (theta_amp <= 0.5)]
              ON.Level1.Operation_mode.Automatic.Double_cycle.container_to_container.Go_down -> Finished1 : [flag_finished_taj==1]
            state To_dock
              entry:mode_balance=0;
              [vyt,vxt,xend,vx_end,vy_end,len] = gen_traj_dock([5,5,15,5,1,1],5,yl0,1,1,m_cont+m_sprider);
              vx_t=vxt; vy_t=vyt;vxend_t=vx_end;vyend_t=vy_end; len_out=len;
              state Go_down
                entry:
                flag_send_traj = 1;
                flag_end_traj=1;
                reset_down =0;
              state Go
                entry:
                flag_send_traj = 1;
                reset_going=0;
              state Finished
                entry:
                flag_semiauto=0;
              (default) -> ON.Level1.Operation_mode.Automatic.Double_cycle.To_dock.Go
              ON.Level1.Operation_mode.Automatic.Double_cycle.To_dock.Go -> ON.Level1.Operation_mode.Automatic.Double_cycle.To_dock.Go_down : [(abs(xend-xl0) <= 0.001) && (theta_amp <= 0.5)]
              ON.Level1.Operation_mode.Automatic.Double_cycle.To_dock.Go_down -> ON.Level1.Operation_mode.Automatic.Double_cycle.To_dock.Finished : [abs(yl0-(5+2.5))<=0.001]
            (default) -> ON.Level1.Operation_mode.Automatic.Double_cycle.To_boat
            ON.Level1.Operation_mode.Automatic.Double_cycle.To_boat.Finished -> container_to_container
            Finished1 -> ON.Level1.Operation_mode.Automatic.Double_cycle.To_dock
          state Simple_cycle
            entry: flag_semiauto = 1;
            flag_end_traj=0;
            flag_send_traj = 0;
            reset_going=0;
            reset_down=0;
            mode_balance = 1;
            state To_boat
              entry:  [vyt,vxt,xend,vx_end,vy_end,len] = gen_traj_boat([5,5,15,5,1,1],xl0,yl0,2,0,m_cont+m_sprider);
              vx_t=vxt; vy_t=vyt;vxend_t=vx_end;vyend_t=vy_end;len_out=len;
              state Go
                entry:
                flag_send_traj = 1;
                reset_going=1;
              state Go_down
                entry:
                flag_send_traj = 1;
                flag_end_traj =1;
                reset_down=1;
              state Finished
                entry:
                flag_end_traj=0;
                flag_send_traj = 0;
              (default) -> ON.Level1.Operation_mode.Automatic.Simple_cycle.To_boat.Go
              ON.Level1.Operation_mode.Automatic.Simple_cycle.To_boat.Go_down -> ON.Level1.Operation_mode.Automatic.Simple_cycle.To_boat.Finished : [flag_finished_taj==1]
              ON.Level1.Operation_mode.Automatic.Simple_cycle.To_boat.Go -> ON.Level1.Operation_mode.Automatic.Simple_cycle.To_boat.Go_down : [(abs(xend-xl0) <= 0.05) && (theta_amp <= 0.5)]
            state To_dock
              entry:mode_balance=0;
              [vyt,vxt,xend,vx_end,vy_end,len] = gen_traj_dock([5,5,15,5,1,1],2,yl0,3,0,m_cont+m_sprider);
              vx_t=vxt; vy_t=vyt;vxend_t=vx_end;vyend_t=vy_end; len_out=len;
              state Go_down
                entry:
                flag_send_traj = 1;
                flag_end_traj=1;
                reset_down =0;
              state Go
                entry:
                flag_send_traj = 1;
                reset_going=0;
              state Finished
                entry:
                flag_semiauto=0;
              (default) -> ON.Level1.Operation_mode.Automatic.Simple_cycle.To_dock.Go
              ON.Level1.Operation_mode.Automatic.Simple_cycle.To_dock.Go -> ON.Level1.Operation_mode.Automatic.Simple_cycle.To_dock.Go_down : [(abs(xend-xl0) <= 0.001) && (theta_amp <= 0.5)]
              ON.Level1.Operation_mode.Automatic.Simple_cycle.To_dock.Go_down -> ON.Level1.Operation_mode.Automatic.Simple_cycle.To_dock.Finished : [flag_finished_taj==1]
            (default) -> ON.Level1.Operation_mode.Automatic.Simple_cycle.To_boat
            ON.Level1.Operation_mode.Automatic.Simple_cycle.To_boat.Finished -> ON.Level1.Operation_mode.Automatic.Simple_cycle.To_dock
          (default) -> Double_cycle
        state Manual
          entry:
          flag_semiauto = 0;
        state Sim_pulsador_aut
        state Sim_pulsador_man
        (default) -> Manual
        Manual -> Sim_pulsador_aut : [switch_mode==1]
        Sim_pulsador_aut -> Automatic : [switch_mode==0]
        Sim_pulsador_man -> Manual : [switch_mode==0]
        Automatic -> Sim_pulsador_man : [switch_mode==1]
      state Load_state [parallel] [commented out]
        state not_loaded [commented out]
          entry:
        state loaded [commented out]
          entry:
        (default) -> not_loaded [commented out]
        not_loaded -> loaded [commented out] : [twistlocks]
        loaded -> not_loaded [commented out] : [~twistlocks]
  (default) -> OFF
  Sim_pulsadorONOFF1 -> OFF : [switch_energy==0]
  OFF -> Sim_pulsadorONOFF : [switch_energy==1]
  ON -> Sim_pulsadorONOFF1 : [switch_energy==1]
  Sim_pulsadorONOFF -> ON : [switch_energy==0]
  data: estado_barco function_input; posx_init function_input; posy_init function_input; posx_end function_input; twistlocks function_input; vdyt function_output; vdxt function_output; x_end function_output; vxt_end function_output; vyt_end function_output; ml function_input; lenght function_output; estado_barco function_input; posx_init function_input; posy_init function_input; posx_end function_input; twistlocks function_input; vdyt function_output; vdxt function_output; x_end function_output; vxt_end function_output; vyt_end function_output; ml function_input; lenght function_output; estado_barco function_input; posx_init function_input; posy_init function_input; posx_end function_input; twistlocks function_input; vdyt function_output; vdxt function_output; x_end function_output; vxt_end function_output; vyt_end function_output; ml function_input; lenght function_output; estado_barco function_input; posx_init function_input; posy_init function_input; posx_end function_input; twistlocks function_input; vdyt function_output; vdxt function_output; x_end function_output; vxt_end function_output; vyt_end function_output; ml function_input; lenght function_output; estado_barco function_input; posx_init function_input; posy_init function_input; posx_end function_input; twistlocks function_input; vdyt function_output; vdxt function_output; x_end function_output; vxt_end function_output; vyt_end function_output; ml function_input; lenght function_output; switch_energy input; switch_mode input; m_cont input; m_sprider input; flag_semiauto output; yl0 input; xl0 input; flag_send_traj output; theta_amp input; xend local double; flag_end_traj output; flag_finished_taj input; go_back input; vyt local size=200000,1; vxt local size=200000,1; vy_end local size=200000,1; vx_end local size=200000,1; balance_switch input; vyend_t output size=200000,1; vy_t output size=200000,1; vxend_t output size=200000,1; vx_t output size=200000,1; len_out output; len local; reset_down output; reset_going output; balancer output; mode_balance output
  function [vdyt,vdxt,x_end,vxt_end,vyt_end,lenght] = gen_traj_boat(estado_barco,posx_init,posy_init,posx_end,twistlocks,ml):
    | function [vdyt,vdxt,x_end,vxt_end,vyt_end,lenght] = gen_traj_boat(estado_barco,posx_init,posy_init,posx_end,twistlocks,ml)
    | coder.extrinsic('gen_traj_to_boat');
    | vdyt = [];
    | vdxt = [];
    | vxt_end =[];
    | vyt_end = [];
    | x_end=0;
    | len=0;
    | coder.varsize('vdyt', [200000 1]);
    | coder.varsize('vdxt', [200000 1]);
    | coder.varsize('vyt_end', [200000 1]);
    | coder.varsize('vxt_end', [200000 1]);
    | [vdyt,vdxt,x_end,vxt_end,vyt_end,lenght]=gen_traj_to_boat(estado_barco,posx_init,posy_init,posx_end,twistlocks, ml);
    | end
  function [vdyt,vdxt,x_end,vxt_end,vyt_end,lenght] = gen_traj_cont_cont(estado_barco,posx_init,posy_init,posx_end,twistlocks,ml):
    | function [vdyt,vdxt,x_end,vxt_end,vyt_end,lenght] = gen_traj_cont_cont(estado_barco,posx_init,posy_init,posx_end,twistlocks,ml)
    | coder.extrinsic('cont_to_cont');
    | vdyt = [];
    | vdxt = [];
    | vxt_end =[];
    | vyt_end = [];
    | x_end=0;
    | coder.varsize('vdyt', [2000000 1]);
    | coder.varsize('vdxt', [2000000 1]);
    | coder.varsize('vyt_end', [2000000 1]);
    | coder.varsize('vxt_end', [2000000 1]);
    | [vdyt,vdxt,x_end,vxt_end,vyt_end,lenght]=cont_to_cont(estado_barco,posx_init,posy_init,posx_end,twistlocks);
    | end
  function [vdyt,vdxt,x_end,vxt_end,vyt_end,lenght] = gen_traj_dock(estado_barco,posx_init,posy_init,posx_end,twistlocks,ml):
    | function [vdyt,vdxt,x_end,vxt_end,vyt_end,lenght] = gen_traj_dock(estado_barco,posx_init,posy_init,posx_end,twistlocks,ml)
    | coder.extrinsic('gen_traj_to_dock');
    | vdyt = [];
    | vdxt = [];
    | vxt_end =[];
    | vyt_end = [];
    | x_end=0;
    | lenght=0;
    | coder.varsize('vdyt', [200000 1]);
    | coder.varsize('vdxt', [200000 1]);
    | coder.varsize('vyt_end', [200000 1]);
    | coder.varsize('vxt_end', [200000 1]);
    | [vdyt,vdxt,x_end,vxt_end,vyt_end,lenght]=gen_traj_to_dock(estado_barco,posx_init,posy_init,posx_end,twistlocks,ml);
    | end
  function [vdyt,vdxt,x_end,vxt_end,vyt_end,lenght] = gen_traj_boat(estado_barco,posx_init,posy_init,posx_end,twistlocks,ml):
    | function [vdyt,vdxt,x_end,vxt_end,vyt_end,lenght] = gen_traj_boat(estado_barco,posx_init,posy_init,posx_end,twistlocks,ml)
    | coder.extrinsic('gen_traj_to_boat');
    | vdyt = [];
    | vdxt = [];
    | vxt_end =[];
    | vyt_end = [];
    | x_end=0;
    | len=0;
    | coder.varsize('vdyt', [200000 1]);
    | coder.varsize('vdxt', [200000 1]);
    | coder.varsize('vyt_end', [200000 1]);
    | coder.varsize('vxt_end', [200000 1]);
    | [vdyt,vdxt,x_end,vxt_end,vyt_end,lenght]=gen_traj_to_boat(estado_barco,posx_init,posy_init,posx_end,twistlocks, ml);
    | end
  function [vdyt,vdxt,x_end,vxt_end,vyt_end,lenght] = gen_traj_dock(estado_barco,posx_init,posy_init,posx_end,twistlocks,ml):
    | function [vdyt,vdxt,x_end,vxt_end,vyt_end,lenght] = gen_traj_dock(estado_barco,posx_init,posy_init,posx_end,twistlocks,ml)
    | coder.extrinsic('gen_traj_to_dock');
    | vdyt = [];
    | vdxt = [];
    | vxt_end =[];
    | vyt_end = [];
    | x_end=0;
    | lenght=0;
    | coder.varsize('vdyt', [200000 1]);
    | coder.varsize('vdxt', [200000 1]);
    | coder.varsize('vyt_end', [200000 1]);
    | coder.varsize('vxt_end', [200000 1]);
    | [vdyt,vdxt,x_end,vxt_end,vyt_end,lenght]=gen_traj_to_dock(estado_barco,posx_init,posy_init,posx_end,twistlocks,ml);
    | end

== matlab function modelofisicocompleto/sending_setpoint_mechanisim/Trajectoria vxt/Subsystem3/Resettable Subsystem/MATLAB Function ==
  data: len_vec input; qd input size=200000,1; cont_i input; cont output; vt output
 function [cont, vt] = fcn(len_vec, qd,cont_i)
 if (cont_i<len_vec)
   cont=cont_i+1;
   vt = qd(cont,1);
 else
  vt = 0;
  cont=inf;
 end
 end

== matlab function modelofisicocompleto/sending_setpoint_mechanisim/Trajectoria vyt/Subsystem3/Resettable Subsystem/MATLAB Function ==
  data: len_vec input; qd input size=200000,1; cont_i input; cont output; vt output
 function [cont, vt] = fcn(len_vec, qd,cont_i)
 if (cont_i<len_vec)
   cont=cont_i+1;
   vt = qd(cont,1);
 else
  vt = 0;
  cont=inf;
 end
 end

== matlab function modelofisicocompleto/sending_setpoint_mechanisim/Trajectoria vyt1/Subsystem3/Resettable Subsystem/MATLAB Function ==
  data: len_vec input; qd input size=200000,1; cont_i input; cont output; vt output
 function [cont, vt] = fcn(len_vec, qd,cont_i)
 if (cont_i<len_vec)
   cont=cont_i+1;
   vt = qd(cont,1);
 else
  vt = 0;
  cont=inf;
 end
 end

== matlab function modelofisicocompleto/sending_setpoint_mechanisim/Trajectoria vyt3/Subsystem3/Resettable Subsystem/MATLAB Function ==
  data: len_vec input; qd input size=200000,1; cont_i input; cont output; vt output
 function [cont, vt] = fcn(len_vec, qd,cont_i)
 if (cont_i<len_vec)
   cont=cont_i+1;
   vt = qd(cont,1);
 else
  vt = 0;
  cont=inf;
 end
 end
